simulink model "k1visetmxt"  (Simulink 8.8)
settings: Solver=ode45  StartTime=0.0  StopTime=10.0  RelTol=1e-3  EnableMultiTasking=on
libraries: cdsIPCx x20, cdsCDI64 x4, cdsCDO64 x4, BIO_CD_ENCODE_MASTER x4, BIO_CD_DECODE_MASTER x4, CHK_DIO x4, cdsAdcx0 x1, cdsCDO32 x1, dac x1, TOWER_MASTER x1, BO_TYPEA_MASTER x1, TESTMON_4CH_MASTER x1
settings Model: SuppressorTable=22 serialization::archive 11 0 3 0 0 0 11 0  Creator=controls  LastModifiedBy=controls
settings DataIOCC: SignalLoggingSaveFormat=Dataset
settings DebuggingCC: UnderspecifiedInitializationDetection=Simplified  MergeDetectMultiDrivingBlocksExec=error  FcnCallInpInsideContextMsg=error  AllowSymbolicDim=off  StateNameClashWarn=none
settings GRTTargetCC: CombineOutputUpdateFcns=on  GRTInterface=off

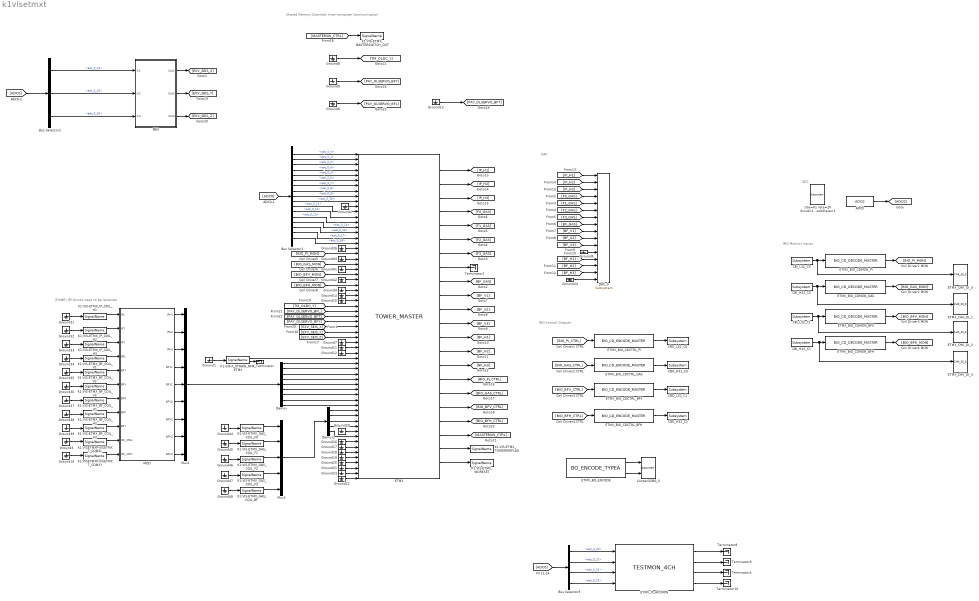
== system k1visetmxt ==
  note: BIO Monitor Inputs
  note: BIO Control Outputs
  note: DAC
  note: ADC
  note: Shared Memory Channels
      | Inner-computer Communication
  note: [FIXME] IPC blocks need to be renamed
  ADC0 : cdsAdcx0/ADC0  Tag=cdsAdc  Description=|
      | type-GSC_16AI64SSA
      | card_num=0
      settings: AttributesFormatString=%<Description>\n%<Tag>
  Bus Selector1 : BusSelector  OutputSignals=adc_0_0,adc_0_1,adc_0_2,adc_0_4,adc_0_5,adc_0_6,adc_0_7,adc_0_8,adc_0_9,adc_0_10,adc_0_11,adc_0_12,adc_0_13,adc_0_14,adc_0_16,adc_0_17,adc_0_18
  Bus Selector2 : BusSelector  OutputSignals=adc_0_24,adc_0_25,adc_0_26
  Bus Selector3 : BusSelector  OutputSignals=adc_0_20,adc_0_21,adc_0_22,adc_0_23
  CBI_H32_C0 : cdsCDI64/Subsystem  Tag=cdsCDI64  Description=card_num=1
      settings: AttributesFormatString=%<Tag>\n%<Description>
  CBI_H32_C1 : cdsCDI64/Subsystem  Tag=cdsCDI64  Description=card_num=3
      settings: AttributesFormatString=%<Tag>\n%<Description>
  CBI_L32_C0 : cdsCDI64/Subsystem  Tag=cdsCDI64  Description=card_num=0
      settings: AttributesFormatString=%<Tag>\n%<Description>
  CBI_L32_C1 : cdsCDI64/Subsystem  Tag=cdsCDI64  Description=card_num=2
      settings: AttributesFormatString=%<Tag>\n%<Description>
  CBO_H32_C0 : cdsCDO64/Subsystem  Tag=cdsCDO64  Description=card_num=1
      settings: AttributesFormatString=%<Tag>\n%<Description>
  CBO_H32_C1 : cdsCDO64/Subsystem  Tag=cdsCDO64  Description=card_num=3
      settings: AttributesFormatString=%<Tag>\n%<Description>
  CBO_L32_C0 : cdsCDO64/Subsystem  Tag=cdsCDO64  Description=card_num=0
      settings: AttributesFormatString=%<Tag>\n%<Description>
  CBO_L32_C1 : cdsCDO64/Subsystem  Tag=cdsCDO64  Description=card_num=2
      settings: AttributesFormatString=%<Tag>\n%<Description>
  Contec32BO_0 : cdsCDO32/Subsystem  Tag=cdsCDO32  Description=Contec32 bit binary output module driver
      settings: AttributesFormatString=%<Tag>
  DAC_0 : dac/Subsystem  Description=|
      | type=GSC_16AO16,
      | card_num=0
      settings: AttributesFormatString=%<Description>
  Demux : Demux  Outputs=9
  Demux1 : Demux  Outputs=5
  ETMX : TOWER_MASTER/TOWER_MASTER
  ETMX_BIO_CDCTRL_BFH : BIO_CD_ENCODE_MASTER/BIO_CD_ENCODE_MASTER
  ETMX_BIO_CDCTRL_BFV : BIO_CD_ENCODE_MASTER/BIO_CD_ENCODE_MASTER
  ETMX_BIO_CDCTRL_GAS : BIO_CD_ENCODE_MASTER/BIO_CD_ENCODE_MASTER
  ETMX_BIO_CDCTRL_PI : BIO_CD_ENCODE_MASTER/BIO_CD_ENCODE_MASTER
  ETMX_BIO_CDMON_BFH : BIO_CD_DECODE_MASTER/BIO_CD_DECODE_MASTER
  ETMX_BIO_CDMON_BFV : BIO_CD_DECODE_MASTER/BIO_CD_DECODE_MASTER
  ETMX_BIO_CDMON_GAS : BIO_CD_DECODE_MASTER/BIO_CD_DECODE_MASTER
  ETMX_BIO_CDMON_PI : BIO_CD_DECODE_MASTER/BIO_CD_DECODE_MASTER
  ETMX_BO_ENCODE : BO_TYPEA_MASTER/BO_ENCODE_TYPEA
  ETMX_CHK_DI_{0..3} (4 alike) : CHK_DIO/CHK_DI_0
  ETMX_IP_ACCMON : TESTMON_4CH_MASTER/TESTMON_4CH
  Ground{1..26,31..39,41..48} (43 alike) : Ground
  K1:GIF-X_STRAIN_RFM_ETMX : cdsIPCx/SignalName  Tag=cdsIPCx_RFM  Description=card=0
      settings: AttributesFormatString=%<Description>\n%<Tag>
  K1:VIS-ETMX_BF_COIL_H1 : cdsIPCx/SignalName  Tag=cdsIPCx_SHMEM  Description=Inter-Process Communication via Shared memory.
      settings: AttributesFormatString=%<Tag>
  K1:VIS-ETMX_BF_COIL_H2 : cdsIPCx/SignalName  Tag=cdsIPCx_SHMEM  Description=Inter-Process Communication via Shared memory.
      settings: AttributesFormatString=%<Tag>
  K1:VIS-ETMX_BF_COIL_H3 : cdsIPCx/SignalName  Tag=cdsIPCx_SHMEM  Description=Inter-Process Communication via Shared memory.
      settings: AttributesFormatString=%<Tag>
  K1:VIS-ETMX_BF_COIL_V1 : cdsIPCx/SignalName  Tag=cdsIPCx_SHMEM  Description=Inter-Process Communication via Shared memory.
      settings: AttributesFormatString=%<Tag>
  K1:VIS-ETMX_BF_COIL_V2 : cdsIPCx/SignalName  Tag=cdsIPCx_SHMEM  Description=Inter-Process Communication via Shared memory.
      settings: AttributesFormatString=%<Tag>
  K1:VIS-ETMX_BF_COIL_V3 : cdsIPCx/SignalName  Tag=cdsIPCx_SHMEM  Description=Inter-Process Communication via Shared memory.
      settings: AttributesFormatString=%<Tag>
  K1:VIS-ETMX_GAS_COIL_BF : cdsIPCx/SignalName  Tag=cdsIPCx_SHMEM  Description=Inter-Process Communication via Shared memory.
      settings: AttributesFormatString=%<Tag>
  K1:VIS-ETMX_GAS_COIL_F{0..3} (4 alike) : cdsIPCx/SignalName  Tag=cdsIPCx_SHMEM  Description=Inter-Process Communication via Shared memory.
      settings: AttributesFormatString=%<Tag>
  K1:VIS-ETMX_IP_COIL_H1 : cdsIPCx/SignalName  Tag=cdsIPCx_SHMEM  Description=Inter-Process Communication via Shared memory.
      settings: AttributesFormatString=%<Tag>
  K1:VIS-ETMX_IP_COIL_H2 : cdsIPCx/SignalName  Tag=cdsIPCx_SHMEM  Description=Inter-Process Communication via Shared memory.
      settings: AttributesFormatString=%<Tag>
  K1:VIS-ETMX_IP_COIL_H3 : cdsIPCx/SignalName  Tag=cdsIPCx_SHMEM  Description=Inter-Process Communication via Shared memory.
      settings: AttributesFormatString=%<Tag>
  K1:VIS-ETMX_MASTERSWITCH_OUT : cdsIPCx/SignalName  Tag=cdsIPCx_SHMEM  Description=Inter-Process Communication via Shared memory.
      settings: AttributesFormatString=%<Tag>
  K1:VIS-ETMX_TOWERWDFLAG : cdsIPCx/SignalName  Tag=cdsIPCx_SHMEM  Description=Inter-Process Communication via Shared memory.
      settings: AttributesFormatString=%<Tag>
  K1:VIS-ETMX_WDRESET : cdsIPCx/SignalName  Tag=cdsIPCx_SHMEM  Description=Inter-Process Communication via Shared memory.
      settings: AttributesFormatString=%<Tag>
  K1:VISETMXP-VISETMXT_COM2L : cdsIPCx/SignalName  Tag=cdsIPCx_SHMEM  Description=Inter-Process Communication via Shared memory.
      settings: AttributesFormatString=%<Tag>
  K1:VISETMXP-VISETMXT_COM2Y : cdsIPCx/SignalName  Tag=cdsIPCx_SHMEM  Description=Inter-Process Communication via Shared memory.
      settings: AttributesFormatString=%<Tag>
  MOD : Subsystem  Tag=top_names
  Mux1 : Mux  Inputs=9
  Mux2 : Mux  Inputs=5
  PEM : Subsystem  Tag=top_names
      settings: AttributesFormatString=%<Tag>
  Terminator{,1,4,8..10} (6 alike) : Terminator
  site=K1 rate=2K dcuid=102 host=k1ex1 specific_cpu=2 adcSlave=1 : cdsParameters/Subsystem  Tag=cdsParameters  Description=|
      | Purpose:                                                                                                                                                                                                                                
      | Provide system parameters to the FE code generator to properly configure the generated EPICS names, rep rate of the FE controller, and the Data Acquisition node ID for proper storage of data from this FE controller.                 
      |                                                                                                                                                                                                                                         
      | Useage:                                                                                                                                                                                                                                 
      | The part NAME field is used to identify the FE parameters. It must be of the form:                                                                                                                                                      
      | site=                                                                                                                                                                                                                                   
      | rate=                                                                                                                                                                                                                                   
      | dcuid=                                                                                                                                                                                                                                  
      |                                                                                                                                                                                                                                         
      | Where:                                                                                                                                                                                                                                  
      | site= argument may be H1, H2, L1, M1, G1, either as a single argument or multiple, for example site=H1,H2. These are the only names allowed. These will become the first two characters of all EPICS and signal names (for example G1:).
      |                                                                                                                                                                                                                                         
      | rate= may be 2K, 16K, 32K, or 64K                                                                                                                                                                                                       
      |                                                                                                                                                                                                                                         
      | dcuid= is site specific ie it must be unique at each site.
      settings: AttributesFormatString=%<Tag>
  wires:
  ADC0/1 -> [ADC0]
  ETMX/4 -> [F0_GAS]
  ETMX/5 -> [F1_GAS]
  ETMX/7 -> [F3_GAS]
  ETMX/6 -> [F2_GAS]
  [BF_H2] -> DAC_0/14
  [BF_V3] -> DAC_0/11
  [BF_H3] -> DAC_0/15
  [BF_V1] -> DAC_0/9
  [BF_H1] -> DAC_0/13
  [BF_V2] -> DAC_0/10
  ETMX/1 -> [IP_H1]
  ETMX/2 -> [IP_H2]
  ETMX/3 -> [IP_H3]
  CBI_H32_C0/1 -> ETMX_CHK_DI_1/1, ETMX_BIO_CDMON_GAS/1
  CBI_L32_C1/1 -> ETMX_CHK_DI_2/1, ETMX_BIO_CDMON_BFV/1
  CBI_L32_C0/1 -> ETMX_CHK_DI_0/1, ETMX_BIO_CDMON_PI/1
  CBI_H32_C1/1 -> ETMX_CHK_DI_3/1, ETMX_BIO_CDMON_BFH/1
  ETMX_BIO_CDCTRL_BFH/1 -> CBO_H32_C1/1
  ETMX_BIO_CDCTRL_PI/1 -> CBO_L32_C0/1
  ETMX_BIO_CDCTRL_GAS/1 -> CBO_H32_C0/1
  ETMX_BIO_CDCTRL_BFV/1 -> CBO_L32_C1/1
  [BIO_PI_CTRL] -> ETMX_BIO_CDCTRL_PI/1
  [BIO_GAS_CTRL] -> ETMX_BIO_CDCTRL_GAS/1
  [BIO_BFV_CTRL] -> ETMX_BIO_CDCTRL_BFV/1
  ETMX_BIO_CDMON_PI/1 -> [BIO_PI_MON]
  ETMX_BIO_CDMON_GAS/1 -> [BIO_GAS_MON]
  ETMX_BIO_CDMON_BFH/1 -> [BIO_BFH_MON]
  ETMX_BIO_CDMON_BFV/1 -> [BIO_BFV_MON]
  [BIO_BFH_CTRL] -> ETMX_BIO_CDCTRL_BFH/1
  [IP_H1] -> DAC_0/1
  [IP_H2] -> DAC_0/2
  [IP_H3] -> DAC_0/3
  [F0_GAS] -> DAC_0/4
  [F1_GAS] -> DAC_0/5
  [F2_GAS] -> DAC_0/6
  [F3_GAS] -> DAC_0/7
  [BF_GAS] -> DAC_0/8
  [ADC0] -> Bus Selector3/1
  Bus Selector3/2 -> ETMX_IP_ACCMON/2  "<adc_0_21>"
  Bus Selector3/1 -> ETMX_IP_ACCMON/1  "<adc_0_20>"
  Bus Selector3/3 -> ETMX_IP_ACCMON/3  "<adc_0_22>"
  Bus Selector3/4 -> ETMX_IP_ACCMON/4  "<adc_0_23>"
  ETMX_IP_ACCMON/3 -> Terminator4/1
  ETMX_IP_ACCMON/4 -> Terminator10/1
  ETMX_IP_ACCMON/1 -> Terminator8/1
  ETMX_IP_ACCMON/2 -> Terminator9/1
  Ground5/1 -> DAC_0/12
  Ground24/1 -> DAC_0/16
  ETMX_BO_ENCODE/1 -> Contec32BO_0/1
  ETMX_BO_ENCODE/2 -> Contec32BO_0/2
  [ADC0] -> Bus Selector1/1
  Ground8/1 -> [TM_OLDC_Y]
  Ground9/1 -> [PAY_OLSERVO_BFY]
  Ground6/1 -> [PAY_OLSERVO_BFL]
  Ground13/1 -> [PAY_OLSERVO_BFT]
  Ground1/1 -> K1:GIF-X_STRAIN_RFM_ETMX/1
  K1:GIF-X_STRAIN_RFM_ETMX/2 -> Terminator/1
  [MASTERSW_CTRL] -> K1:VIS-ETMX_MASTERSWITCH_OUT/1
  [ADC0] -> Bus Selector2/1
  Bus Selector2/1 -> PEM/1(In1)  "<adc_0_24>"
  Bus Selector2/2 -> PEM/2(In2)  "<adc_0_25>"
  Bus Selector2/3 -> PEM/3(In3)  "<adc_0_26>"
  PEM/1(Out1) -> [EXV_SEIS_X]
  PEM/2(Out2) -> [EXV_SEIS_Y]
  PEM/3(Out3) -> [EXV_SEIS_Z]
  Ground31/1 -> K1:VIS-ETMX_IP_COIL_H1/1
  Ground32/1 -> K1:VIS-ETMX_IP_COIL_H2/1
  Ground33/1 -> K1:VIS-ETMX_IP_COIL_H3/1
  Ground34/1 -> K1:VIS-ETMX_BF_COIL_V1/1
  Ground35/1 -> K1:VIS-ETMX_BF_COIL_V2/1
  Ground36/1 -> K1:VIS-ETMX_BF_COIL_V3/1
  Ground37/1 -> K1:VIS-ETMX_BF_COIL_H1/1
  Ground38/1 -> K1:VIS-ETMX_BF_COIL_H2/1
  Ground39/1 -> K1:VIS-ETMX_BF_COIL_H3/1
  Mux1/1 -> Demux/1
  K1:VIS-ETMX_IP_COIL_H1/1 -> MOD/1(IPL)
  K1:VIS-ETMX_IP_COIL_H2/1 -> MOD/2(IPT)
  K1:VIS-ETMX_IP_COIL_H3/1 -> MOD/3(IPY)
  K1:VIS-ETMX_BF_COIL_V1/1 -> MOD/4(BFL)
  K1:VIS-ETMX_BF_COIL_V2/1 -> MOD/5(BFT)
  K1:VIS-ETMX_BF_COIL_V3/1 -> MOD/6(BFV)
  K1:VIS-ETMX_BF_COIL_H1/1 -> MOD/7(BFR)
  K1:VIS-ETMX_BF_COIL_H2/1 -> MOD/8(BFP)
  K1:VIS-ETMX_BF_COIL_H3/1 -> MOD/9(BFY)
  MOD/1(IPH1) -> Mux1/1
  MOD/2(IPH2) -> Mux1/2
  MOD/3(IPH3) -> Mux1/3
  MOD/4(BFV1) -> Mux1/4
  MOD/5(BFV2) -> Mux1/5
  MOD/6(BFV3) -> Mux1/6
  MOD/7(BFH1) -> Mux1/7
  MOD/8(BFH2) -> Mux1/8
  MOD/9(BFH3) -> Mux1/9
  K1:VISETMXP-VISETMXT_COM2L/1 -> MOD/10(ISC_MNL)
  K1:VIS-ETMX_GAS_COIL_F0/1 -> Mux2/1
  K1:VIS-ETMX_GAS_COIL_F1/1 -> Mux2/2
  K1:VIS-ETMX_GAS_COIL_F2/1 -> Mux2/3
  K1:VIS-ETMX_GAS_COIL_F3/1 -> Mux2/4
  K1:VIS-ETMX_GAS_COIL_BF/1 -> Mux2/5
  Ground44/1 -> K1:VIS-ETMX_GAS_COIL_F0/1
  Ground45/1 -> K1:VIS-ETMX_GAS_COIL_F1/1
  Ground46/1 -> K1:VIS-ETMX_GAS_COIL_F2/1
  Ground47/1 -> K1:VIS-ETMX_GAS_COIL_F3/1
  Ground48/1 -> K1:VIS-ETMX_GAS_COIL_BF/1
  Mux2/1 -> Demux1/1
  K1:VISETMXP-VISETMXT_COM2Y/1 -> MOD/11(ISC_MNY)
  Ground3/1 -> K1:VISETMXP-VISETMXT_COM2L/1
  Ground10/1 -> K1:VISETMXP-VISETMXT_COM2Y/1
  Bus Selector1/1 -> ETMX/1  "<adc_0_0>"
  Bus Selector1/2 -> ETMX/2  "<adc_0_1>"
  Bus Selector1/3 -> ETMX/3  "<adc_0_2>"
  Bus Selector1/4 -> ETMX/4  "<adc_0_4>"
  Bus Selector1/5 -> ETMX/5  "<adc_0_5>"
  Bus Selector1/6 -> ETMX/6  "<adc_0_6>"
  Bus Selector1/7 -> ETMX/7  "<adc_0_7>"
  Bus Selector1/8 -> ETMX/8  "<adc_0_8>"
  Bus Selector1/9 -> ETMX/9  "<adc_0_9>"
  Bus Selector1/10 -> ETMX/10  "<adc_0_10>"
  Bus Selector1/11 -> ETMX/12  "<adc_0_11>"
  Ground2/1 -> ETMX/11
  [BIO_PI_MON] -> ETMX/20
  [BIO_GAS_MON] -> ETMX/22
  Ground43/1 -> ETMX/21
  Ground41/1 -> ETMX/23
  [BIO_BFV_MON] -> ETMX/24
  Ground42/1 -> ETMX/25
  Bus Selector1/17 -> ETMX/18  "<adc_0_18>"
  Bus Selector1/16 -> ETMX/17  "<adc_0_17>"
  Bus Selector1/15 -> ETMX/16  "<adc_0_16>"
  Bus Selector1/14 -> ETMX/15  "<adc_0_14>"
  Bus Selector1/13 -> ETMX/14  "<adc_0_13>"
  Bus Selector1/12 -> ETMX/13  "<adc_0_12>"
  Ground22/1 -> ETMX/63
  Ground23/1 -> ETMX/62
  Ground21/1 -> ETMX/61
  Ground25/1 -> ETMX/60
  Ground19/1 -> ETMX/59
  Ground18/1 -> ETMX/58
  Ground17/1 -> ETMX/57
  Ground16/1 -> ETMX/56
  Demux1/5 -> ETMX/55
  Demux1/4 -> ETMX/53
  Demux1/3 -> ETMX/52
  Demux1/2 -> ETMX/51
  Demux1/1 -> ETMX/50
  Ground20/1 -> ETMX/54
  Demux/9 -> ETMX/49
  Demux/8 -> ETMX/48
  Demux/7 -> ETMX/47
  Demux/6 -> ETMX/46
  Demux/5 -> ETMX/45
  Demux/4 -> ETMX/44
  Demux/3 -> ETMX/43
  Demux/2 -> ETMX/42
  Demux/1 -> ETMX/41
  K1:GIF-X_STRAIN_RFM_ETMX/1 -> ETMX/40
  Ground7/1 -> ETMX/37
  Ground11/1 -> ETMX/38
  Ground12/1 -> ETMX/39
  [EXV_SEIS_Z] -> ETMX/36
  [EXV_SEIS_Y] -> ETMX/35
  [EXV_SEIS_X] -> ETMX/34
  [PAY_OLSERVO_BFY] -> ETMX/33
  [PAY_OLSERVO_BFT] -> ETMX/32
  [PAY_OLSERVO_BFL] -> ETMX/31
  [TM_OLDC_Y] -> ETMX/30
  Ground15/1 -> ETMX/29
  Ground14/1 -> ETMX/28
  Ground4/1 -> ETMX/27
  [BIO_BFH_MON] -> ETMX/26
  Ground26/1 -> ETMX/19
  ETMX/22 -> K1:VIS-ETMX_WDRESET/1
  ETMX/21 -> K1:VIS-ETMX_TOWERWDFLAG/1
  ETMX/20 -> [MASTERSW_CTRL]
  ETMX/19 -> [BIO_BFH_CTRL]
  ETMX/18 -> [BIO_BFV_CTRL]
  ETMX/17 -> [BIO_GAS_CTRL]
  ETMX/16 -> [BIO_PI_CTRL]
  ETMX/13 -> [BF_H1]
  ETMX/14 -> [BF_H2]
  ETMX/15 -> [BF_H3]
  ETMX/10 -> [BF_V1]
  ETMX/11 -> [BF_V2]
  ETMX/12 -> [BF_V3]
  ETMX/9 -> [BF_GAS]
  ETMX/8 -> Terminator1/1

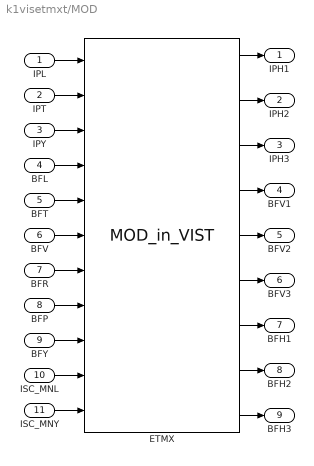
== system k1visetmxt/MOD ==
  IPL : Inport
  IPT : Inport  Port=2
  IPY : Inport  Port=3
  BFL : Inport  Port=4
  BFT : Inport  Port=5
  BFV : Inport  Port=6
  BFR : Inport  Port=7
  BFP : Inport  Port=8
  BFY : Inport  Port=9
  ISC_MNL : Inport  Port=10
  ISC_MNY : Inport  Port=11
  ETMX : VIS_LIB/MODAL/MOD_in_VIST  Tag=top_names
  IPH1 : Outport
  IPH2 : Outport  Port=2
  IPH3 : Outport  Port=3
  BFV1 : Outport  Port=4
  BFV2 : Outport  Port=5
  BFV3 : Outport  Port=6
  BFH1 : Outport  Port=7
  BFH2 : Outport  Port=8
  BFH3 : Outport  Port=9
  wires:
  IPL/1 -> ETMX/1
  IPT/1 -> ETMX/2
  IPY/1 -> ETMX/3
  BFL/1 -> ETMX/4
  BFT/1 -> ETMX/5
  BFV/1 -> ETMX/6
  BFR/1 -> ETMX/7
  BFP/1 -> ETMX/8
  BFY/1 -> ETMX/9
  ETMX/1 -> IPH1/1
  ETMX/2 -> IPH2/1
  ETMX/3 -> IPH3/1
  ETMX/4 -> BFV1/1
  ETMX/5 -> BFV2/1
  ETMX/6 -> BFV3/1
  ETMX/7 -> BFH1/1
  ETMX/8 -> BFH2/1
  ETMX/9 -> BFH3/1
  ISC_MNL/1 -> ETMX/10
  ISC_MNY/1 -> ETMX/11

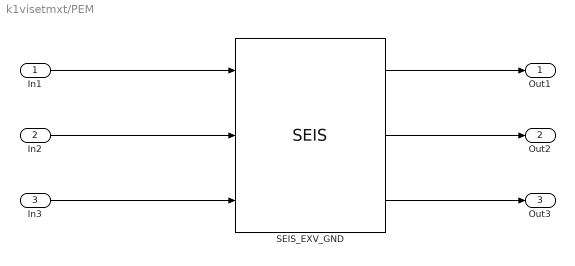
== system k1visetmxt/PEM ==
  In1 : Inport
  In2 : Inport  Port=2
  In3 : Inport  Port=3
  SEIS_EXV_GND : seis/SEIS
  Out1 : Outport
  Out2 : Outport  Port=2
  Out3 : Outport  Port=3
  wires:
  SEIS_EXV_GND/1 -> Out1/1
  SEIS_EXV_GND/2 -> Out2/1
  SEIS_EXV_GND/3 -> Out3/1
  In1/1 -> SEIS_EXV_GND/1
  In2/1 -> SEIS_EXV_GND/2
  In3/1 -> SEIS_EXV_GND/3
